simulink library "lib_EMachine_2017a"  (R2017b)
settings: Solver=VariableStepAuto  StartTime=0.0  StopTime=10.0  RelTol=1e-3
undefined symbols (not defined in the file): EngineTorqueReal, mot, motor_Trq, t_amb, time, tloop
libraries: simulink x5, autolibmappedmotor x3
(part 2 of 3)

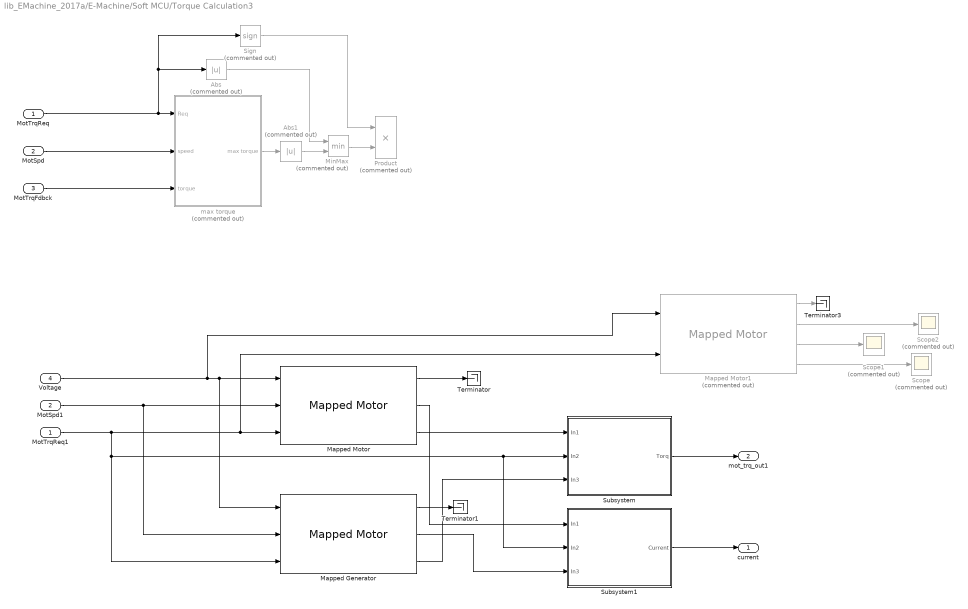
== system lib_EMachine_2017a/E-Machine/Soft MCU/Torque Calculation3 ==
  MotTrqReq : Inport
  MotSpd : Inport  Port=2
  MotTrqFdbck : Inport  Port=3
  Voltage : Inport  Port=4
  Abs : Abs  Commented=on  ZeroCross=off
  Abs1 : Abs  Commented=on  ZeroCross=off
  Mapped Generator : autolibmappedmotor/Mapped Motor  port_config=Speed  param_by=Maximum torque and power  w_t=[ 0 375 750 800 ]  T_t=[0.09 0.08 0.07 0]  torque_max=300  power_max=70000  Tc=0.02  param_loss=Tabulated efficiency data  eff=100  w_eff=375  T_eff=0.08  Piron=0  Pbase=0  w_eff_bp=[0 500 1000 1500 2000 2500 3000 3500 4000 4500 5000 5500 6000 6500 7000]  T_eff_bp=[25 50 75 100 112 125 150 165 175 200 225 250 262 275 300]  losses_table=[1.49 1.67 2.21 3.10; 0.42 0.69 1.14 2.03; 0.06 0.24 0.78 1.68; 0.42 0.69 1.14 2.03; 1.49 1.67 2.21 3.10]  efficiency_table=mot.plant.init.geneff_trq.map  J=5e-6  b=1e-5  omega_o=0  T_t_extended=[0 0.07 0.08 0.09 0.08 0.07 0]  w_t_extended=[-800 -750 -375 0 375 750 800]  KLossIron=0  KLossCopper=0  x_w_eff_vec=[-7000 -6500 -6000 -5500 -5000 -4500 -4000 -3500 -3000 -2500 -2000 -1500 -1000 -500 0 500 1000 1500 2000 2500 3000 3500 4000 4500 5000 5500 6000 6500 7000]  x_T_eff_vec=[-300 -275 -262 -250 -225 -200 -175 -165 -150 -125 -112 -100 -75 -50 -25 25 50 75 100 112 125 150 165 175 200 225 250 262 275 300]  x_losses_mat=[2566666.66666667 607894.736842105 517282.051282051 493589.743589743 393750 307317.073170732 233333.333333333 220000 200000 119318.181818182 106909.090909091 95454.5454545455 58333.3333333334 30434.7826086956 213888.888888889 96250 28000 52500 84000 94080 105000 168000 184800 196000 252000 315000 385000 403480 462000 1155000;2383333.33333333 290988.372093023 277232.558139535 221590.909090909 199431.818181818 144444.444444445 98913.0434782608 93260.8695652173 84782.6086956521 70652.1739130434 46468.085106383 41489.3617021276 42391.3043478261 28260.8695652174 198611.111111111 89375 26000 39000 39000 43680 65000 78000 85800 91000 130000 175500 195000 238420 250250 1072500;2200000 183333.333333333 174666.666666667 166666.666666667 150000 76595.744680851 67021.2765957447 63191.4893617021 57446.8085106383 47872.3404255319 42893.6170212766 38297.8723404255 50000 40909.0909090909 183333.333333333 82500 36000 45000 36000 40320 45000 53999.9999999999 59399.9999999999 62999.9999999999 71999.9999999999 135000 150000 157200 165000 990000;2016666.66666667 96542.5531914893 91978.7234042553 87765.9574468085 78989.3617021276 70212.7659574468 61436.1702127659 57925.5319148936 52659.5744680851 43882.9787234042 39319.1489361702 35106.3829787234 45833.3333333334 37500 168055.555555556 75625 33000 41250 33000 36960 41250 49499.9999999999 54449.9999999999 57749.9999999999 65999.9999999999 74249.9999999999 82499.9999999999 86459.9999999999 90749.9999999999 907500;1833333.33333333 87765.9574468085 83617.0212765957 79787.2340425532 71808.5106382979 63829.7872340425 55851.0638297872 52659.5744680851 47872.3404255319 39893.6170212766 35744.6808510638 109756.097560976 41666.6666666667 34090.9090909091 152777.777777778 68750 30000 37500 90000 33600 37500 45000 49499.9999999999 52499.9999999999 59999.9999999999 67499.9999999999 74999.9999999999 78599.9999999999 82499.9999999999 825000;1650000 78989.3617021276 75255.3191489361 71808.5106382979 64627.6595744681 57446.8085106383 50265.9574468085 47393.6170212766 43085.1063829787 35904.2553191489 43826.0869565217 50000 46022.7272727273 36627.9069767442 137500 61875 31500 40500 45000 40320 33750 40500 44550 47250 53999.9999999999 60749.9999999999 67499.9999999999 70739.9999999999 74249.9999999999 742500;1466666.66666667 733333.333333333 698666.666666667 86956.5217391304 57446.8085106383 51063.829787234 44680.8510638298 42127.6595744681 52173.9130434782 43478.2608695652 49777.7777777778 44444.4444444445 48837.2093023256 50000 122222.222222222 55000 40000 42000 40000 44800 40000 48000 39600 42000 48000 53999.9999999999 80000 419200 440000 660000;1283333.33333333 641666.666666667 611333.333333333 97222.2222222223 50265.9574468085 44680.8510638298 53260.8695652174 50217.3913043478 45652.1739130435 48611.1111111111 43555.5555555556 47727.2727272728 57621.9512195122 49358.9743589743 106944.444444444 48125 38500 47250 42000 39200 43750 42000 46200 49000 42000 47250 87500 366800 385000 577500;1100000 550000 524000 500000 75000 38297.8723404255 45652.1739130435 43043.4782608695 39130.4347826087 41666.6666666667 37333.3333333334 33333.3333333334 52777.7777777778 42307.6923076923 91666.6666666667 41250 33000 42750 30000 33600 37500 36000 39600 42000 36000 67500 300000 314400 330000 495000;916666.666666667 458333.333333333 436666.666666667 416666.666666667 375000 333333.333333333 27925.5319148936 35869.5652173913 32608.6956521739 34722.2222222222 31111.1111111111 40697.6744186047 43981.4814814815 39473.6842105263 76388.8888888889 34375 30000 35625 35000 28000 31250 30000 33000 26250 200000 225000 250000 262000 275000 412500;733333.333333333 366666.666666667 349333.333333333 333333.333333333 300000 266666.666666667 233333.333333333 45000 19148.9361702128 27777.7777777778 24888.8888888889 38095.2380952381 35185.1851851852 35135.1351351351 61111.1111111111 27500 26000 28500 32000 22400 25000 18000 39600 140000 160000 180000 200000 209600 220000 330000;550000 275000 262000 250000 225000 200000 175000 15797.8723404255 ...(+5787 chars)]
      settings: SourceProductName=Powertrain Blockset  SourceProductBaseCode=PW
  Mapped Motor : autolibmappedmotor/Mapped Motor  port_config=Speed  param_by=Maximum torque and power  w_t=[ 0 375 750 800 ]  T_t=[0.09 0.08 0.07 0]  torque_max=337  power_max=80000  Tc=0.02  param_loss=Tabulated efficiency data  eff=100  w_eff=375  T_eff=0.08  Piron=0  Pbase=0  w_eff_bp=[0 500 1000 1500 2000 2500 3000 3500 4000 4500 5000 5500 6000 6500 7000]  T_eff_bp="[88.2  98.7 106.4 119 132.2 155.6 175.6 208 243 295.3 328 329 333.5 334.5 335]"  losses_table=[1.49 1.67 2.21 3.10; 0.42 0.69 1.14 2.03; 0.06 0.24 0.78 1.68; 0.42 0.69 1.14 2.03; 1.49 1.67 2.21 3.10]  efficiency_table=mot.plant.init.moteff_trq.map  J=5e-6  b=1e-5  omega_o=0  T_t_extended=[0 0.07 0.08 0.09 0.08 0.07 0]  w_t_extended=[-800 -750 -375 0 375 750 800]  KLossIron=0  KLossCopper=0  x_w_eff_vec=[-7000 -6500 -6000 -5500 -5000 -4500 -4000 -3500 -3000 -2500 -2000 -1500 -1000 -500 0 500 1000 1500 2000 2500 3000 3500 4000 4500 5000 5500 6000 6500 7000]  x_T_eff_vec=[-335 -334.5 -333.5 -329 -328 -295.3 -243 -208 -175.6 -155.6 -132.2 -119 -106.4 -98.7 -88.2 88.2 98.7 106.4 119 132.2 155.6 175.6 208 243 295.3 328 329 333.5 334.5 335]  x_losses_mat=[1563333.33333333 381174.418604651 318340.909090909 314045.454545455 313090.909090909 281877.272727273 231954.545454546 161777.777777778 136577.777777778 94713.0434782608 80469.5652173912 72434.7826086956 31033.3333333334 60078.2608695652 411600 246960 55272 29792 66640 74032 87136 122920 145600 204120 248052 275520 276360 280140 327810 938000;1451666.66666667 296488.636363637 240861.111111111 185956.52173913 185391.304347826 166908.695652174 137347.826086956 117565.217391304 99252.1739130434 87947.8260869565 74721.7391304347 85944.4444444445 94309.090909091 104438.372093023 382200 229320 89817 82992 77350 68744 80912 91312 108160 126360 153556 170560 171080 216775 260910 871000;1340000 273681.818181818 222333.333333333 171652.173913043 171130.434782609 73825.0000000001 126782.608695652 108521.739130435 91617.3913043478 81182.6086956521 68973.9130434782 79333.3333333334 87054.5454545455 96404.6511627907 352800 211680 82908 76608 71400 63456 74688 84288 99840 116640 70872.0000000001 157440 157920 200100 240840 804000;1228333.33333333 1226500 203805.555555556 157347.826086956 115148.936170213 67672.9166666668 55687.5000000001 73021.2765957447 83982.6086956521 74417.3913043478 63226.0869565217 72722.2222222222 79800.0000000001 88370.9302325582 323400 194040 75999 70224 65450 58168 68464 77264 68639.9999999999 53460.0000000001 64966.0000000001 108240 144760 183425 735900 737000;1116666.66666667 1115000 1111666.66666667 182777.777777778 104680.85106383 61520.8333333334 50625.0000000001 66382.9787234042 56042.5531914893 67652.1739130434 57478.2608695652 66111.1111111111 72545.4545454546 80337.2093023256 294000 176400 69090 63840 59500 52880 62240 52679.9999999999 62399.9999999999 48600 59060.0000000001 98399.9999999999 164500 667000 669000 670000;1005000 1003500 1000500 987000 984000 115552.173913043 95086.9565217391 81391.304347826 68713.0434782608 60886.9565217391 66100 59500 65290.9090909091 97496.3414634146 264600 158760 79947 57456 53550 59490 56016 63216 74880 87480 106308 590400 592200 600300 602100 603000;893333.333333333 892000 889333.333333333 877333.333333333 145777.777777778 131244.444444445 84521.7391304347 72347.8260869565 61078.2608695652 54121.7391304347 58755.5555555556 58831.4606741573 69283.7209302326 98700 235200 141120 78960 59584 52360 52880 49792 56192 66560 77760 118120 131200 526400 533600 535200 536000;781666.666666667 780500 778166.666666667 767666.666666667 765333.333333333 689033.333333333 567000 485333.333333333 53443.4782608695 60511.1111111111 57187.6404494382 56795.4545454546 70933.3333333333 97434.6153846153 205800 123480 75999 59584 49980 50897 54460 49168 291200 340200 413420 459200 460600 466900 468300 469000;670000 669000 667000 658000 656000 590600 486000 416000 351200 51866.6666666667 49017.9775280899 58116.2790697675 65378.313253012 93505.2631578948 176400 105840 71064 54264 49980 43626 46680 210720 249600 291600 354360 393600 394800 400200 401400 402000;558333.333333333 557500 555833.333333333 548333.333333333 546666.666666667 492166.666666667 405000 346666.666666667 292666.666666667 259333.333333333 53802.3255813954 56666.6666666667 62395.061728395 110858.695652174 147000 88200 76492.5 50540 47600 46270 155600 175600 208000 243000 295300 328000 329000 333500 334500 335000;446666.666666667 446000 444666.666666667 438666.666666667 437333.333333333 393733.333333333 324000 277333.333333333 234133.333333333 207466.666666667 43041.8604651163 45333.3333333333 60020.5128205128 88686.9565217391 117600 70560 61194 46816 38080 37016 124480 140480 166400 194400 236240 262400 263200 266800 267600 268000;335000 334500 333500 329000 328000 295300 243000 208000 175600 155600 32281.3953488372 34000 50400 79719.2307692308 88200 52920 51817.5 38304 28560 27762 93360 105360 124800 145800 177180 196800 197400 200100 200700 201000;223333.333333333 223000 222333.333333333 219333.333333333 218666.666666667 196866.666666667 162000 138666.666666667 117066.666666667 103733.333333333 21520.9302325581 22666.6666666667 ...(+4913 chars)]
      settings: SourceProductName=Powertrain Blockset  SourceProductBaseCode=PW
  Mapped Motor1 : autolibmappedmotor/Mapped Motor  Commented=on  port_config=Torque  param_by=Maximum torque and power  w_t=[ 0 375 750 800 ]  T_t=[0.09 0.08 0.07 0]  torque_max=337  power_max=70000  Tc=0.02  param_loss=Tabulated efficiency data  eff=100  w_eff=375  T_eff=0.08  Piron=0  Pbase=0  w_eff_bp=[0 500 1000 1500 2000 2500 3000 3500 4000 4500 5000 5500 6000 6500 7000]  T_eff_bp="[88.2  98.7 106.4 119 132.2 155.6 175.6 208 243 295.3 328 329 333.5 334.5 335]"  losses_table=[1.49 1.67 2.21 3.10; 0.42 0.69 1.14 2.03; 0.06 0.24 0.78 1.68; 0.42 0.69 1.14 2.03; 1.49 1.67 2.21 3.10]  efficiency_table=mot.plant.init.moteff_trq.map  J=5e-6  b=1e-5  omega_o=0  T_t_extended=[0 0.07 0.08 0.09 0.08 0.07 0]  w_t_extended=[-800 -750 -375 0 375 750 800]  KLossIron=0  KLossCopper=0  x_w_eff_vec=[-7000 -6500 -6000 -5500 -5000 -4500 -4000 -3500 -3000 -2500 -2000 -1500 -1000 -500 0 500 1000 1500 2000 2500 3000 3500 4000 4500 5000 5500 6000 6500 7000]  x_T_eff_vec=[-335 -334.5 -333.5 -329 -328 -295.3 -243 -208 -175.6 -155.6 -132.2 -119 -106.4 -98.7 -88.2 88.2 98.7 106.4 119 132.2 155.6 175.6 208 243 295.3 328 329 333.5 334.5 335]  x_losses_mat=[1563333.33333333 381174.418604651 318340.909090909 314045.454545455 313090.909090909 281877.272727273 231954.545454546 161777.777777778 136577.777777778 94713.0434782608 80469.5652173912 72434.7826086956 31033.3333333334 60078.2608695652 411600 246960 55272 29792 66640 74032 87136 122920 145600 204120 248052 275520 276360 280140 327810 938000;1451666.66666667 296488.636363637 240861.111111111 185956.52173913 185391.304347826 166908.695652174 137347.826086956 117565.217391304 99252.1739130434 87947.8260869565 74721.7391304347 85944.4444444445 94309.090909091 104438.372093023 382200 229320 89817 82992 77350 68744 80912 91312 108160 126360 153556 170560 171080 216775 260910 871000;1340000 273681.818181818 222333.333333333 171652.173913043 171130.434782609 73825.0000000001 126782.608695652 108521.739130435 91617.3913043478 81182.6086956521 68973.9130434782 79333.3333333334 87054.5454545455 96404.6511627907 352800 211680 82908 76608 71400 63456 74688 84288 99840 116640 70872.0000000001 157440 157920 200100 240840 804000;1228333.33333333 1226500 203805.555555556 157347.826086956 115148.936170213 67672.9166666668 55687.5000000001 73021.2765957447 83982.6086956521 74417.3913043478 63226.0869565217 72722.2222222222 79800.0000000001 88370.9302325582 323400 194040 75999 70224 65450 58168 68464 77264 68639.9999999999 53460.0000000001 64966.0000000001 108240 144760 183425 735900 737000;1116666.66666667 1115000 1111666.66666667 182777.777777778 104680.85106383 61520.8333333334 50625.0000000001 66382.9787234042 56042.5531914893 67652.1739130434 57478.2608695652 66111.1111111111 72545.4545454546 80337.2093023256 294000 176400 69090 63840 59500 52880 62240 52679.9999999999 62399.9999999999 48600 59060.0000000001 98399.9999999999 164500 667000 669000 670000;1005000 1003500 1000500 987000 984000 115552.173913043 95086.9565217391 81391.304347826 68713.0434782608 60886.9565217391 66100 59500 65290.9090909091 97496.3414634146 264600 158760 79947 57456 53550 59490 56016 63216 74880 87480 106308 590400 592200 600300 602100 603000;893333.333333333 892000 889333.333333333 877333.333333333 145777.777777778 131244.444444444 84521.7391304347 72347.8260869565 61078.2608695652 54121.7391304347 58755.5555555556 58831.4606741573 69283.7209302326 98700 235200 141120 78960 59584 52360 52880 49792 56192 66560 77760 118120 131200 526400 533600 535200 536000;781666.666666667 780500 778166.666666667 767666.666666667 765333.333333333 689033.333333333 567000 485333.333333333 53443.4782608695 60511.1111111111 57187.6404494382 56795.4545454546 70933.3333333333 97434.6153846153 205800 123480 75999 59584 49980 50897 54460 49168 291200 340200 413420 459200 460600 466900 468300 469000;670000 669000 667000 658000 656000 590600 486000 416000 351200 51866.6666666667 49017.9775280899 58116.2790697675 65378.313253012 93505.2631578948 176400 105840 71064 54264 49980 43626 46680 210720 249600 291600 354360 393600 394800 400200 401400 402000;558333.333333333 557500 555833.333333333 548333.333333333 546666.666666667 492166.666666667 405000 346666.666666667 292666.666666667 259333.333333333 53802.3255813954 56666.6666666667 62395.061728395 110858.695652174 147000 88200 76492.5 50540 47600 46270 155600 175600 208000 243000 295300 328000 329000 333500 334500 335000;446666.666666667 446000 444666.666666667 438666.666666667 437333.333333333 393733.333333333 324000 277333.333333333 234133.333333333 207466.666666667 43041.8604651163 45333.3333333333 60020.5128205128 88686.9565217391 117600 70560 61194 46816 38080 37016 124480 140480 166400 194400 236240 262400 263200 266800 267600 268000;335000 334500 333500 329000 328000 295300 243000 208000 175600 155600 32281.3953488372 34000 50400 79719.2307692308 88200 52920 51817.5 38304 28560 27762 93360 105360 124800 145800 177180 196800 197400 200100 200700 201000;223333.333333333 223000 222333.333333333 219333.333333333 218666.666666667 196866.666666667 162000 138666.666666667 117066.666666667 103733.333333333 21520.9302325581 22666.6666666667 ...(+4913 chars)]
      settings: SourceProductName=Powertrain Blockset  SourceProductBaseCode=PW
  MinMax : MinMax  Commented=on  Inputs=2  ZeroCross=off
  MotSpd1 : InportShadow  Port=2
  MotTrqReq1 : InportShadow
  Product : Product  Commented=on
  Scope : Scope  Commented=on
  Scope1 : Scope  Commented=on
  Scope2 : Scope  Commented=on
  Sign : Signum  Commented=on  ZeroCross=off
  Subsystem : Subsystem
  Subsystem1 : Subsystem
  Terminator : Terminator
  Terminator1 : Terminator
  Terminator3 : Terminator
  "max torque " : Subsystem  Commented=on
  current : Outport
  mot_trq_out1 : Outport  Port=2
  wires:
  Mapped Motor1/4 -> Scope/1
  Mapped Motor1/1 -> Terminator3/1
  Mapped Motor1/2 -> Scope2/1
  Mapped Motor1/3 -> Scope1/1
  Subsystem1/1(Current) -> current/1
  Subsystem/1(Torq) -> mot_trq_out1/1
  Mapped Generator/2 -> Subsystem1/3(In3)
  Mapped Motor/2 -> Subsystem1/1(In1)
  Mapped Generator/3 -> Subsystem/3(In3)
  Mapped Motor/3 -> Subsystem/1(In1)
  Mapped Generator/1 -> Terminator1/1
  Mapped Motor/1 -> Terminator/1
  Voltage/1 -> Mapped Motor/1, Mapped Generator/1, Mapped Motor1/1
  MotSpd1/1 -> Mapped Motor/2, Mapped Generator/2
  MotTrqReq1/1 -> Mapped Motor/3, Mapped Motor1/2, Subsystem/2(In2), Subsystem1/2(In2), Mapped Generator/3
  MotTrqFdbck/1 -> "max torque "/3(torque)
  Abs1/1 -> MinMax/2
  Abs/1 -> MinMax/1
  MinMax/1 -> Product/2
  Sign/1 -> Product/1
  MotTrqReq/1 -> "max torque "/1(Req), Abs/1, Sign/1
  MotSpd/1 -> "max torque "/2(speed)
  "max torque "/1(max torque) -> Abs1/1

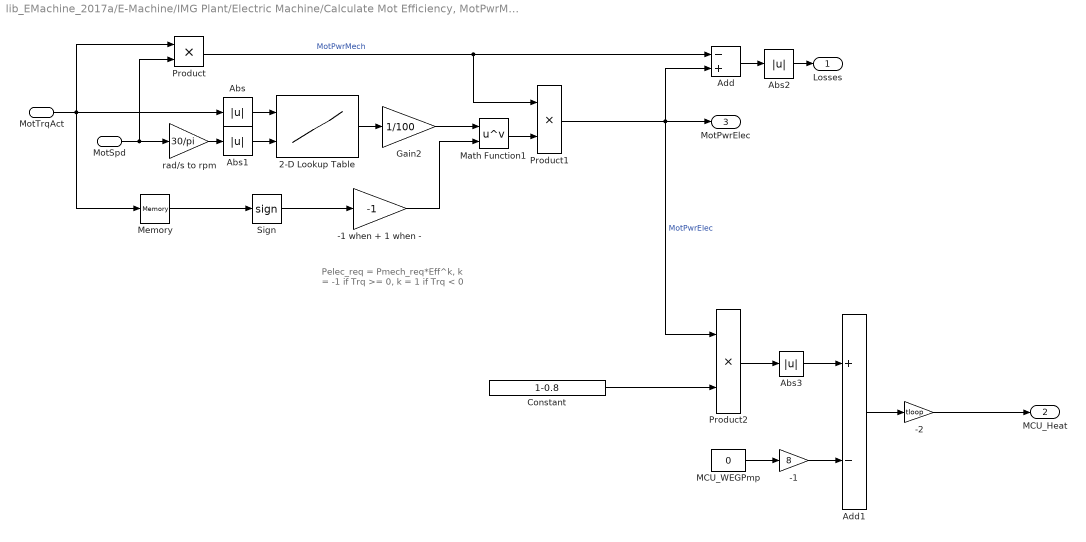
== system lib_EMachine_2017a/E-Machine/IMG Plant/Electric Machine/Calculate Mot Efficiency, MotPwrMech, and, MotPwrElec1 ==
  note: Pelec_req = Pmech_req*Eff^k,
      | k = -1 if Trq >= 0,
      | k = 1 if Trq < 0
  MotSpd : Inport
  MotTrqAct : Inport  Port=2
  -1 : Gain  Gain=8
  "-1 when + 1 when - " : Gain  Gain=-1
  -2 : Gain  Gain=tloop
  2-D Lookup Table : Lookup_n-D  BreakpointsForDimension1=mot.plant.init.eff_trq.idx2_trq  BreakpointsForDimension2=mot.plant.init.eff_trq.idx1_spd  Table=mot.plant.init.eff_trq.map  InternalRulePriority=Speed  RndMeth=Simplest  InputSameDT=on
  Abs{,1..3} (4 alike) : Abs
  Add : Sum  Inputs=-+
  Add1 : Sum  Inputs=+-
  Constant : Constant  Value=1-0.8
  Gain2 : Gain  Gain=1/100
  MCU_WEGPmp : Constant  Value=0
  Math Function1 : Math  Operator=pow  SaturateOnIntegerOverflow=on
  Memory : Memory
  Product : Product
  Product1 : Product
  Product2 : Product
  Sign : Signum
  rad/s to rpm : Gain  Gain=30/pi
  Losses : Outport
  MCU_Heat : Outport  Port=2
  MotPwrElec : Outport  Port=3
  wires:
  rad/s to rpm/1 -> Abs1/1
  Abs1/1 -> 2-D Lookup Table/2
  Sign/1 -> "-1 when + 1 when - "/1
  Abs/1 -> 2-D Lookup Table/1
  Gain2/1 -> Math Function1/1
  2-D Lookup Table/1 -> Gain2/1
  Product1/1 -> MotPwrElec/1, Product2/1, Add/2  "MotPwrElec"
  Product/1 -> Add/1, Product1/1  "MotPwrMech"
  MotTrqAct/1 -> Memory/1, Product/1, Abs/1
  MotSpd/1 -> Product/2, rad/s to rpm/1
  "-1 when + 1 when - "/1 -> Math Function1/2
  Abs2/1 -> Losses/1
  Add/1 -> Abs2/1
  Math Function1/1 -> Product1/2
  Memory/1 -> Sign/1
  Constant/1 -> Product2/2
  Product2/1 -> Abs3/1
  Abs3/1 -> Add1/1
  MCU_WEGPmp/1 -> -1/1
  Add1/1 -> -2/1
  -1/1 -> Add1/2
  -2/1 -> MCU_Heat/1

== system lib_EMachine_2017a/E-Machine/IMG Plant/Electric Machine/MotTrqExcessTrigger1 ==
  In1 : Inport
  Bias : Bias  Bias=55
  Bias1 : Bias  Bias=25
  Constant : Constant  Value=0
  Multiport Switch : MultiPortSwitch  DataPortOrder=Zero-based contiguous
  Terminator : Terminator
  Out1 : Outport
  tag scope: MotTrqExcessTrig=global
  wires:
  [MotTrqExcessTrig] -> Terminator/1
  Multiport Switch/1 -> Out1/1
  Bias/1 -> Multiport Switch/4
  In1/1 -> Multiport Switch/2, Bias/1, Bias1/1
  Bias1/1 -> Multiport Switch/3
  Constant/1 -> [MotTrqExcessTrig], Multiport Switch/1

== system lib_EMachine_2017a/E-Machine/IMG Plant/Electric Machine/Thermal1 ==
  Losses : Inport
  MCU_heat : Inport  Port=2
  MotInv_loop : Subsystem
  Motor Thermal : Subsystem  Commented=on
  MCU_temp_C : Outport
  motor_temp : Outport  Port=2
  wires:
  MCU_heat/1 -> MotInv_loop/2(In2)
  Losses/1 -> MotInv_loop/1(In1)  "[W]"
  MotInv_loop/1(Out1) -> MCU_temp_C/1
  MotInv_loop/2(Out2) -> motor_temp/1

== system lib_EMachine_2017a/E-Machine/IMG Plant/Electric Machine/Torque Calculation1 ==
  MotSpd : Inport
  MotTrqCmd : Inport  Port=2
  Abs : Abs
  Abs1 : Abs
  Memory : Memory
  MinMax : MinMax  Inputs=2
  Product : Product
  Sign : Signum
  "max torque " : Subsystem
  mot_trq_out : Outport
  wires:
  "max torque "/1(max torque) -> Abs1/1
  MotSpd/1 -> "max torque "/2(speed)
  Sign/1 -> Product/1
  MinMax/1 -> Product/2
  Abs/1 -> MinMax/1
  Abs1/1 -> MinMax/2
  Memory/1 -> mot_trq_out/1
  MotTrqCmd/1 -> "max torque "/1(cmd), Sign/1, Abs/1
  Product/1 -> Memory/1

== system lib_EMachine_2017a/E-Machine/IMG Plant/Electric Machine/non-zero division1 ==
  note: original idea from Phil Sharer - ANL
      | original formula: u[1]\(u[2]+eps)*(u[2]!=0)
      | changes done by Gerald ZINI (dgey) - ANL (05\02\2001)
  note: (u[2]==0) is true then returns 1, thus (u[2]+(u[2]==0)) is equal to 0+1=1
  note: if u[2] == 0, then output == 0:
  note: (u[2]!=0) is false then returns 0
  note: and finally, the expression is: (u[1] \ 1) * 0 = 0
  note: (u[2]==0) is false then returns 0, thus (u[2]+(u[2]==0)) is equal to u[2]+0=u[2]
  note: if u[2] != 0, then output == u[1]\u[2]:
  note: (u[2]!=0) is true then returns 1
  note: and finally, the expression is: (u[1] \ u[2]) * 1 = u[1] \ u[2]
  In1 : Inport
  In2 : Inport  Port=2
  Fcn : Fcn  Expr=u[1]/(u[2]+(u[2]==0))*(u[2]!=0)
  Mux : Mux  Inputs=2
  Out1 : Outport
  wires:
  Mux/1 -> Fcn/1
  In1/1 -> Mux/1
  Fcn/1 -> Out1/1
  In2/1 -> Mux/2

== system lib_EMachine_2017a/E-Machine/IMG Plant2/Calculate Mot Efficiency, MotPwrMech, and, MotPwrElec/Lower Limit ==
  In1 : Inport
  Constant3 : Constant  Value=Lolimit
  MinMax : MinMax  Function=max  Inputs=2
  Out1 : Outport
  wires:
  In1/1 -> MinMax/1
  Constant3/1 -> MinMax/2
  MinMax/1 -> Out1/1

== system lib_EMachine_2017a/E-Machine/IMG Plant2/Calculate Mot Efficiency, MotPwrMech, and, MotPwrElec/MCUOverTemp Fault ==
  In1 : Inport
  Gain : Gain  Gain=3
  Switch : Switch  Threshold=1
  Out1 : Outport
  wires:
  In1/1 -> Switch/3, Gain/1
  [MCUOverTemp] -> Switch/2
  Gain/1 -> Switch/1
  Switch/1 -> Out1/1

== system lib_EMachine_2017a/E-Machine/IMG Plant2/Motor_Plant/Efficiency Calcs ==
  Speed_rpm : Inport
  Torq_cmd_Nm : Inport  Port=2
  Batt_volt : Inport  Port=3
  Abs1 : Abs
  Constant : Constant
  Constant1 : Constant  Value=0
  Current_consum : Product  Inputs=*/
  Efficiency Map : Lookup_n-D  BreakpointsForDimension1=mot.map.trqindex  BreakpointsForDimension2=mot.map.spdindex  Table=mot.map.eff  InternalRulePriority=Speed  RndMeth=Simplest  InputSameDT=on
  Electrical power motoring : Product  Inputs=*//
  Electrical power regen : Product  Inputs=***
  Gain : Gain  Gain=2*3.14/60
  Gain1 : Gain  Gain=-1
  MCU_eff : Constant  Value=0.97
  Mech_power : Product  Inputs=**
  MinMax : MinMax  Function=max  Inputs=2
  MinMax1 : MinMax  Function=max  Inputs=2
  Saturation : Saturate  UpperLimit=400  LowerLimit=-400
  Switch : Switch  Criteria=u2 > Threshold
  Switch1 : Switch  Criteria=u2 > Threshold  Threshold=100
  min_eff : Constant  Value=0.1
  Mot_current : Outport
  Mech_power_W : Outport  Port=2
  Elec_power_W : Outport  Port=3
  wires:
  Speed_rpm/1 -> Efficiency Map/2, Gain/1
  Torq_cmd_Nm/1 -> Mech_power/2, Abs1/1, Switch/2
  Electrical power regen/1 -> Switch/3
  MinMax/1 -> Electrical power motoring/2, Electrical power regen/2
  Current_consum/1 -> Gain1/1
  Saturation/1 -> Mot_current/1  "Mot_current_A"
  Gain/1 -> Mech_power/1
  Batt_volt/1 -> Switch1/2, MinMax1/1
  Abs1/1 -> Efficiency Map/1
  Mech_power/1 -> Electrical power motoring/1, Electrical power regen/1, Mech_power_W/1  "Mech_power_W"
  MCU_eff/1 -> Electrical power regen/3, Electrical power motoring/3
  Electrical power motoring/1 -> Switch/1
  min_eff/1 -> MinMax/2
  Switch1/1 -> Elec_power_W/1, Current_consum/1  "Elec_power_W"
  Efficiency Map/1 -> MinMax/1
  MinMax1/1 -> Current_consum/2
  Constant/1 -> MinMax1/2
  Gain1/1 -> Saturation/1  "Mot_current_A"
  Switch/1 -> Switch1/1  "Elec_power_W"
  Constant1/1 -> Switch1/3

== system lib_EMachine_2017a/E-Machine/IMG Plant2/Thermal/Motor Thermal ==
  In1 : Inport
  Add1 : Sum  Inputs=+-
  Add2 : Sum
  Divide : Product  Inputs=*/
  Lower Limit : Subsystem  mask{Lolimit=t_amb+20}
      mask prompts: Lolimit "Lower Limit"
  Memory1 : Memory
  Motor Mass : Constant  Value=mot.plant.init.motor_mass
  Product : Product  RndMeth=Zero
  "Pump " : Constant  Value=0
  Specific Heat Cap Aluminum : Constant  Value=mot.plant.init.specific_heat
  tloop : Gain  Gain=tloop
  Out1 : Outport
  wires:
  Specific Heat Cap Aluminum/1 -> Product/2  "J/kg*K"
  Product/1 -> Divide/2
  Memory1/1 -> Add2/2
  Add2/1 -> Lower Limit/1(In1)
  Lower Limit/1(Out1) -> Out1/1, Memory1/1
  Divide/1 -> Add2/1
  tloop/1 -> Divide/1  "J"
  Motor Mass/1 -> Product/1  "kg"
  "Pump "/1 -> Add1/2
  In1/1 -> Add1/1
  Add1/1 -> tloop/1

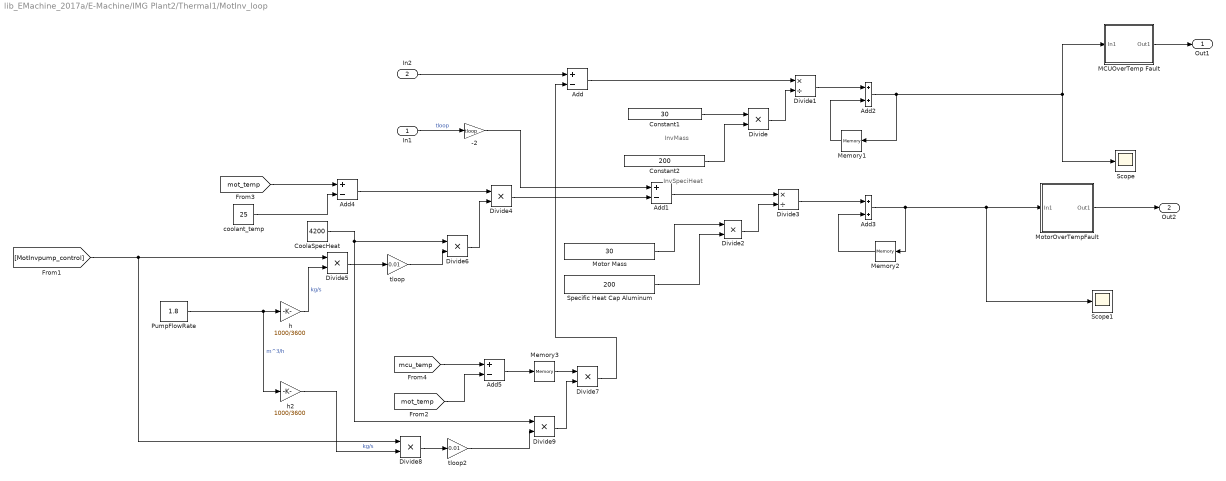
== system lib_EMachine_2017a/E-Machine/IMG Plant2/Thermal1/MotInv_loop ==
  note: InvSpeciHeat
  note: InvMass
  In1 : Inport
  In2 : Inport  Port=2
  -2 : Gain  Gain=tloop
  Add{,1,4..5} (4 alike) : Sum  Inputs=+-
  Add2 : Sum
  Add3 : Sum
  Constant1 : Constant  Value=30
  Constant2 : Constant  Value=200
  CoolaSpecHeat : Constant  Value=4200
  Divide{,2,4..9} (8 alike) : Product  Inputs=**
  Divide1 : Product  Inputs=*/
  Divide3 : Product  Inputs=*/
  MCUOverTemp Fault : Subsystem
  Memory1 : Memory  InitialCondition=25
  Memory2 : Memory  InitialCondition=25
  Memory3 : Memory
  Motor Mass : Constant  Value=30
  MotorOverTempFault : Subsystem
  PumpFlowRate : Constant  Value=1.8
  Scope : Scope
  Scope1 : Scope
  Specific Heat Cap Aluminum : Constant  Value=200
  coolant_temp : Constant  Value=25
  h : Gain  Gain=1000/3600
  h2 : Gain  Gain=1000/3600
  tloop : Gain  Gain=0.01
  tloop2 : Gain  Gain=0.01
  Out1 : Outport
  Out2 : Outport  Port=2
  wires:
  Add1/1 -> Divide3/1
  Memory1/1 -> Add2/2
  coolant_temp/1 -> Add4/2
  Divide/1 -> Divide1/2
  Specific Heat Cap Aluminum/1 -> Divide2/2
  Constant1/1 -> Divide/1
  Add/1 -> Divide1/1
  Memory2/1 -> Add3/2
  Add4/1 -> Divide4/1
  Add3/1 -> Scope1/1, MotorOverTempFault/1(In1), Memory2/1
  Divide6/1 -> Divide4/2
  Divide3/1 -> Add3/1
  Divide5/1 -> tloop/1
  Add2/1 -> MCUOverTemp Fault/1(In1), Scope/1, Memory1/1
  Divide2/1 -> Divide3/2
  Constant2/1 -> Divide/2
  Motor Mass/1 -> Divide2/1
  Divide1/1 -> Add2/1
  Divide7/1 -> Add/2
  h/1 -> Divide5/2  "kg/s"
  tloop/1 -> Divide6/2
  CoolaSpecHeat/1 -> Divide6/1, Divide9/1
  PumpFlowRate/1 -> h2/1, h/1  "m^3/h"
  h2/1 -> Divide8/2  "kg/s"
  Divide9/1 -> Divide7/2
  Divide8/1 -> tloop2/1
  tloop2/1 -> Divide9/2
  Divide4/1 -> Add1/2
  Add5/1 -> Memory3/1
  Memory3/1 -> Divide7/1
  MCUOverTemp Fault/1(Out1) -> Out1/1
  MotorOverTempFault/1(Out1) -> Out2/1
  [mot_temp] -> Add4/1
  [mcu_temp] -> Add5/1
  [mot_temp] -> Add5/2
  In1/1 -> -2/1  "tloop"
  In2/1 -> Add/1
  -2/1 -> Add1/1
  [MotInvpump_control] -> Divide8/1, Divide5/1

== system lib_EMachine_2017a/E-Machine/IMG Plant2/Thermal1/Motor Thermal ==
  In1 : Inport
  Add1 : Sum  Inputs=+-
  Add2 : Sum
  Divide : Product  Inputs=*/
  Lower Limit : Subsystem  mask{Lolimit=t_amb+20}
      mask prompts: Lolimit "Lower Limit"
  Memory1 : Memory
  Motor Mass : Constant  Value=mot.plant.init.motor_mass
  Product : Product  RndMeth=Zero
  "Pump " : Constant  Value=0
  Specific Heat Cap Aluminum : Constant  Value=mot.plant.init.specific_heat
  tloop : Gain  Gain=tloop
  Out1 : Outport
  wires:
  Specific Heat Cap Aluminum/1 -> Product/2  "J/kg*K"
  Product/1 -> Divide/2
  Memory1/1 -> Add2/2
  Add2/1 -> Lower Limit/1(In1)
  Lower Limit/1(Out1) -> Out1/1, Memory1/1
  Divide/1 -> Add2/1
  tloop/1 -> Divide/1  "J"
  Motor Mass/1 -> Product/1  "kg"
  "Pump "/1 -> Add1/2
  In1/1 -> Add1/1
  Add1/1 -> tloop/1

== system lib_EMachine_2017a/E-Machine/IMG Plant2/Torque Calculation/electric machine filter ==
  trq : Inport
  Interval Test : simulink/Logic and Bit Operations/Interval Test  IntervalClosedRight=on  uplimit=0.5  IntervalClosedLeft=on  lowlimit=-0.5  OutDataTypeStr=boolean
  Switch : Switch  Threshold=0.5
  electric machine time response : TransferFcn  Denominator=[mot.plant.init.time_response 1]
  filtered : Outport
  wires:
  electric machine time response/1 -> Switch/3
  Interval Test/1 -> Switch/2
  trq/1 -> Interval Test/1, electric machine time response/1, Switch/1
  Switch/1 -> filtered/1

== system lib_EMachine_2017a/E-Machine/IMG Plant2/Torque Calculation/max torque  ==
  cmd : Inport
  speed : Inport  Port=2
  Memory : Memory
  Peak trq max - Motoring : Lookup  InputValues=mot.plant.init.regen.trq_max.idx1_spd  Table=mot.plant.init.motor.trq_max.map  LookUpMeth=Interpolation-Use End Values  SaturateOnIntegerOverflow=on
  Peak trq max - Regen : Lookup  InputValues=mot.plant.init.regen.trq_max.idx1_spd  Table=mot.plant.init.regen.trq_max.map  LookUpMeth=Interpolation-Use End Values  SaturateOnIntegerOverflow=on
  Switch1 : Switch  SaturateOnIntegerOverflow=on
  rad/s  to RPM : Gain  Gain=30/pi
  max torque : Outport
  wires:
  Peak trq max - Motoring/1 -> Switch1/1
  speed/1 -> rad/s  to RPM/1
  cmd/1 -> Switch1/2
  Switch1/1 -> max torque/1
  Memory/1 -> Peak trq max - Motoring/1, Peak trq max - Regen/1
  rad/s  to RPM/1 -> Memory/1
  Peak trq max - Regen/1 -> Switch1/3

== system lib_EMachine_2017a/E-Machine/Soft MCU/Subsystem/MCU_RollingAliveCnt ==
  Counter Free-Running : simulink/Sources/Counter Free-Running  NumBits=4  tsamp=-1
  Out1 : Outport
  wires:
  Counter Free-Running/1 -> Out1/1  "MCURollingAliveCnt [0 1 2 3]"

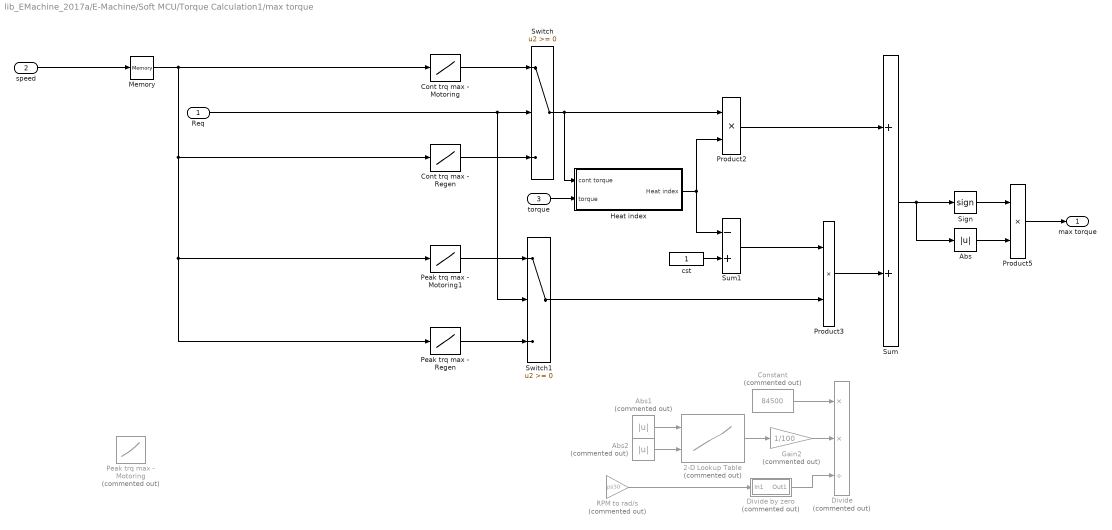
== system lib_EMachine_2017a/E-Machine/Soft MCU/Torque Calculation1/max torque  ==
  Req : Inport
  speed : Inport  Port=2
  torque : Inport  Port=3
  2-D Lookup Table : Lookup_n-D  Commented=on  BreakpointsForDimension1=mot.plant.init.eff_trq.idx2_trq  BreakpointsForDimension2=mot.plant.init.eff_trq.idx1_spd  Table=mot.plant.init.eff_trq.map  InternalRulePriority=Speed  RndMeth=Simplest  InputSameDT=on
  Abs : Abs  SaturateOnIntegerOverflow=on
  Abs1 : Abs  Commented=on
  Abs2 : Abs  Commented=on
  Constant : Constant  Commented=on  Value=84500
  Cont trq max - Motoring : Lookup  InputValues=mot.plant.init.motor.trq_cont.idx1_spd  Table=mot.plant.init.motor.trq_cont.map  LookUpMeth=Interpolation-Use End Values  SaturateOnIntegerOverflow=on
  Cont trq max - Regen : Lookup  InputValues=mot.plant.init.regen.trq_cont.idx1_spd  Table=mot.plant.init.regen.trq_cont.map  LookUpMeth=Interpolation-Use End Values  SaturateOnIntegerOverflow=on
  Divide : Product  Commented=on  Inputs=**/
  Divide by zero : Subsystem  Commented=on
  Gain2 : Gain  Commented=on  Gain=1/100
  Heat index : Subsystem
  Memory : Memory
  Peak trq max - Motoring : Lookup  Commented=on  InputValues=mot.plant.init.regen.trq_max.idx1_spd  Table=mot.plant.init.motor.trq_max.map  LookUpMeth=Interpolation-Use End Values  SaturateOnIntegerOverflow=on
  Peak trq max - Motoring1 : Lookup  InputValues=mot.plant.init.regen.trq_max.idx1_spd  Table=mot.plant.init.motor.trq_max.map  LookUpMeth=Interpolation-Use End Values  SaturateOnIntegerOverflow=on
  Peak trq max - Regen : Lookup  InputValues=mot.plant.init.regen.trq_max.idx1_spd  Table=mot.plant.init.regen.trq_max.map  LookUpMeth=Interpolation-Use End Values  SaturateOnIntegerOverflow=on
  Product2 : Product  SaturateOnIntegerOverflow=on  InputSameDT=on  OutDataTypeStr=Inherit: Same as first input
  Product3 : Product  SaturateOnIntegerOverflow=on  InputSameDT=on  OutDataTypeStr=Inherit: Same as first input
  Product5 : Product  SaturateOnIntegerOverflow=on  InputSameDT=on  OutDataTypeStr=Inherit: Same as first input
  RPM to rad/s : Gain  Commented=on  Gain=pi/30
  Sign : Signum
  Sum : Sum  SaturateOnIntegerOverflow=on  InputSameDT=on  OutDataTypeStr=Inherit: Same as first input
  Sum1 : Sum  Inputs=-+  SaturateOnIntegerOverflow=on  InputSameDT=on  OutDataTypeStr=Inherit: Same as first input
  Switch : Switch  SaturateOnIntegerOverflow=on
  Switch1 : Switch  SaturateOnIntegerOverflow=on
  cst : Constant
  max torque : Outport
  wires:
  Peak trq max - Motoring1/1 -> Switch1/1
  Divide by zero/1(Out1) -> Divide/3
  Req/1 -> Switch1/2, Switch/2
  Gain2/1 -> Divide/2
  2-D Lookup Table/1 -> Gain2/1
  Abs1/1 -> 2-D Lookup Table/1
  Abs2/1 -> 2-D Lookup Table/2
  RPM to rad/s/1 -> Divide by zero/1(In1)
  Constant/1 -> Divide/1
  speed/1 -> Memory/1
  Memory/1 -> Peak trq max - Regen/1, Peak trq max - Motoring1/1, Cont trq max - Regen/1, Cont trq max - Motoring/1
  Sign/1 -> Product5/1
  Product5/1 -> max torque/1
  Sum/1 -> Sign/1, Abs/1
  Abs/1 -> Product5/2
  torque/1 -> Heat index/2(torque)
  Cont trq max - Motoring/1 -> Switch/1
  Cont trq max - Regen/1 -> Switch/3
  Peak trq max - Regen/1 -> Switch1/3
  Switch/1 -> Product2/1, Heat index/1(cont torque)
  Switch1/1 -> Product3/2
  Product2/1 -> Sum/1
  Sum1/1 -> Product3/1
  Product3/1 -> Sum/2
  cst/1 -> Sum1/2
  Heat index/1(Heat index) -> Sum1/1, Product2/2
